simulink model "udp_com"  (R2021b)
settings: Solver=FixedStepAuto  StartTime=0.0  StopTime=10  RelTol=1e-3
libraries: dspnetwork x2, slrealtimeutilitieslib x1, sldrtlib x1
settings Model: Creator=cihad  LastModifiedBy=xls
settings SolverCC: AlgebraicLoopSolver=TrustRegion
settings DataIOCC: ReturnWorkspaceOutputs=off
settings DebuggingCC: SFMachineParentedDataDiag=warning  ArithmeticOperatorsInVariantConditions=warning
settings SFSimCC: SimUseLocalCustomCode=off  CustomCodeUndefinedFunction=UseInterfaceOnly
settings RTWCC: RTWUseLocalCustomCode=off

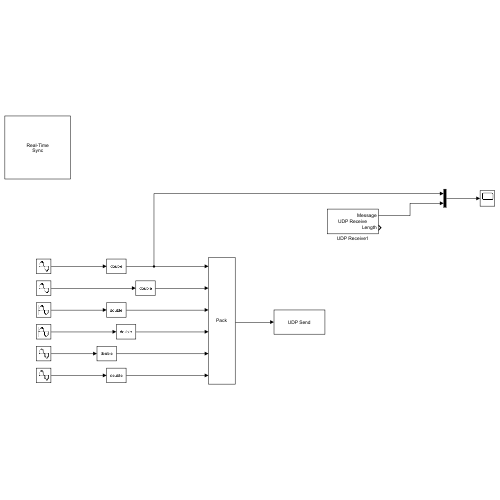
[thumbnail: Simulink's stored preview of the top-level diagram]
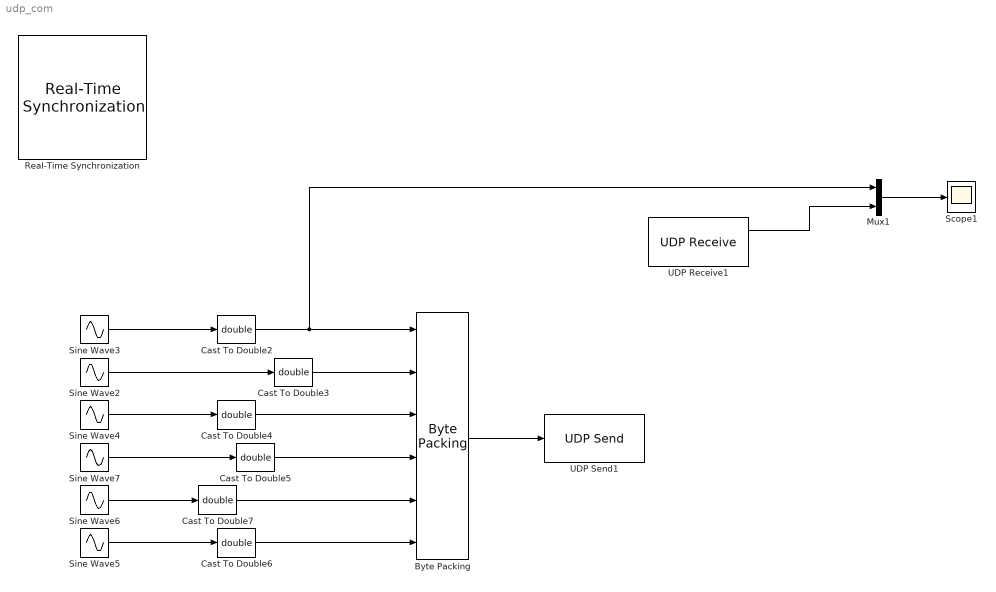
== system udp_com ==
  Byte Packing : slrealtimeutilitieslib/Byte Packing  MaskPackedDataType=double  MaskUnpackedDataTypes={'double','double','double','double','double','double'}  MaskAlignment=1
  Cast To Double{2..7} (6 alike) : DataTypeConversion  OutDataTypeStr=double
  Mux1 : Mux  Inputs=2
  Real-Time Synchronization : sldrtlib/Real-Time Synchronization  SampleTime=0.01  MaxMissedTicks=100000  ShowMissedTicks=off  YieldWhenWaiting=off
  Scope1 : Scope
  Sine Wave2 : Sin  Amplitude=2  SampleTime=0.01
  Sine Wave3 : Sin  SampleTime=0.01
  Sine Wave4 : Sin  Amplitude=3  SampleTime=0.01
  Sine Wave5 : Sin  Amplitude=6  SampleTime=0.01
  Sine Wave6 : Sin  Amplitude=51  SampleTime=0.01
  Sine Wave7 : Sin  Amplitude=4  SampleTime=0.01
  UDP Receive1 : dspnetwork/UDP Receive  localURL='0.0.0.0'  localPort=26000  remoteURL='0.0.0.0'  remotePort=-1  recvBufferSize=8192  dims=1  signalDatatype=double  isComplex=off  isVarSize=off  showBlockingTime=off  blockingTime=0  sampletime=0.001  blockPlatform=[]
  UDP Send1 : dspnetwork/UDP Send  remoteURL='127.0.0.1'  remotePort=23333  localURL='0.0.0.0'  localPortSource=Automatically determine  localPort=-1  sendBufferSize=8192  sampletime=-1  blockPlatform=[]  separateLengthPort=0
  wires:
  Mux1/1 -> Scope1/1
  Cast To Double2/1 -> Mux1/1, Byte Packing/1
  UDP Receive1/1 -> Mux1/2
  Sine Wave2/1 -> Cast To Double3/1
  Sine Wave3/1 -> Cast To Double2/1
  Sine Wave4/1 -> Cast To Double4/1
  Sine Wave5/1 -> Cast To Double6/1
  Sine Wave6/1 -> Cast To Double7/1
  Sine Wave7/1 -> Cast To Double5/1
  Byte Packing/1 -> UDP Send1/1
  Cast To Double3/1 -> Byte Packing/2
  Cast To Double6/1 -> Byte Packing/6
  Cast To Double5/1 -> Byte Packing/4
  Cast To Double7/1 -> Byte Packing/5
  Cast To Double4/1 -> Byte Packing/3
